simulink model "dxl_xm430"  (Simulink 7.6)
settings: Solver=FixedStepDiscrete  StartTime=0.0  StopTime=Inf  RelTol=1e-3
libraries: rpi_blkst x1
settings Model: Creator=jacques  LastModifiedBy=jacques
settings OptimizationCC: OptimizeModelRefInitCode=on  LifeSpan=1
settings HardwareCC: ProdLargestAtomicInteger=Long  ProdLargestAtomicFloat=Double  ProdEndianess=LittleEndian  ProdHWDeviceType=ARM Compatible->ARM 11
settings RTWCC: SystemTargetFile=ert_rpi.tlc  TemplateMakefile=ert_rpi.tmf  PostCodeGenCommand=postGenFunc(buildInfo)  Description=RTW Embedded Coder RPI target  ProcessScript=ert_rpi_make_rtw_hook
settings CodeAppCC: IgnoreCustomStorageClasses=off
settings STFCustomTargetCC: ModelReferenceCompliant=off  CombineOutputUpdateFcns=on  ERTCustomFileBanners=on  SupportNonInlinedSFcns=off  SystemTargetFile=ert_rpi.tlc
settings ERTTargetCC: MultiwordLength=2048  ModelReferenceCompliant=off  ParMdlRefBuildCompliant=off  CompOptLevelCompliant=off  ERTFirstTimeCompliant=off  SupportContinuousTime=on  ModelStepFunctionPrototypeControlCompliant=off  CPPClassGenCompliant=off  ExtMode=on  ExtModeMexArgs='130.79.73.46'  InlinedParameterPlacement=NonHierarchical  ERTCustomFileTemplate=ert_rpi_file_process.tlc  ConvertIfToSwitch=off

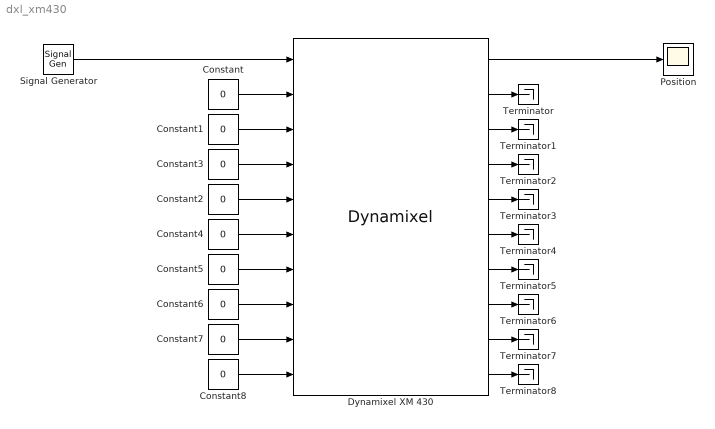
== system dxl_xm430 ==
  Constant{,1..8} (9 alike) : Constant  Value=0  SampleTime=0.01
  Dynamixel XM 430 : rpi_blkst/Dynamixel  SystemSampleTime=-1  rpi_mask_Ts=0.01  rpi_mask_portname=0  rpi_mask_baudrate=1000000  rpi_mask_startid=1  rpi_mask_nbid=1  rpi_mask_proto=2  rpi_mask_write_addr=116  rpi_mask_write_length=4  rpi_mask_read_addr=132  rpi_mask_read_length=4  rpi_mask_read_sign=1  rpi_mask_init1_addr=1  rpi_mask_init1_length=1  rpi_mask_init1_data=4  rpi_mask_init2_addr=80  rpi_mask_init2_length=2  rpi_mask_init2_data=0  rpi_mask_init3_addr=82  rpi_mask_init3_length=2  rpi_mask_init3_data=0  rpi_mask_init4_addr=84  rpi_mask_init4_length=2  rpi_mask_init4_data=800  rpi_mask_init5_addr=88  rpi_mask_init5_length=2  rpi_mask_init5_data=0  rpi_mask_init6_addr=90  rpi_mask_init6_length=2  rpi_mask_init6_data=0  rpi_mask_init7_addr=65  rpi_mask_init7_length=1  rpi_mask_init7_data=1  rpi_mask_init8_addr=64  rpi_mask_init8_length=1  rpi_mask_init8_data=1  rpi_mask_halt1_addr=64  rpi_mask_halt1_length=1  rpi_mask_halt1_data=0  rpi_mask_halt2_addr=65  rpi_mask_halt2_length=1  rpi_mask_halt2_data=0
  Position : Scope
  Signal Generator : SignalGenerator  WaveForm=square  Amplitude=500
  Terminator{,1..8} (9 alike) : Terminator
  wires:
  Dynamixel XM 430/2 -> Terminator/1
  Dynamixel XM 430/3 -> Terminator1/1
  Dynamixel XM 430/4 -> Terminator2/1
  Dynamixel XM 430/5 -> Terminator3/1
  Dynamixel XM 430/6 -> Terminator4/1
  Dynamixel XM 430/7 -> Terminator5/1
  Dynamixel XM 430/8 -> Terminator6/1
  Dynamixel XM 430/9 -> Terminator7/1
  Dynamixel XM 430/10 -> Terminator8/1
  Constant/1 -> Dynamixel XM 430/2
  Constant1/1 -> Dynamixel XM 430/3
  Constant3/1 -> Dynamixel XM 430/4
  Constant2/1 -> Dynamixel XM 430/5
  Constant4/1 -> Dynamixel XM 430/6
  Constant5/1 -> Dynamixel XM 430/7
  Constant6/1 -> Dynamixel XM 430/8
  Constant7/1 -> Dynamixel XM 430/9
  Constant8/1 -> Dynamixel XM 430/10
  Dynamixel XM 430/1 -> Position/1
  Signal Generator/1 -> Dynamixel XM 430/1
